simulink model "Properties_Controller_Tank1_Primitives"  (R2012b)
settings: Solver=FixedStepDiscrete  StartTime=0.0  StopTime=10.0  FixedStep=0.1  RelTol=1e-3
settings Model: Creator=Kerianne  LastModifiedBy=Kerianne
settings DataIOCC: SaveFormat=Structure
settings OptimizationCC: InlineParams=on

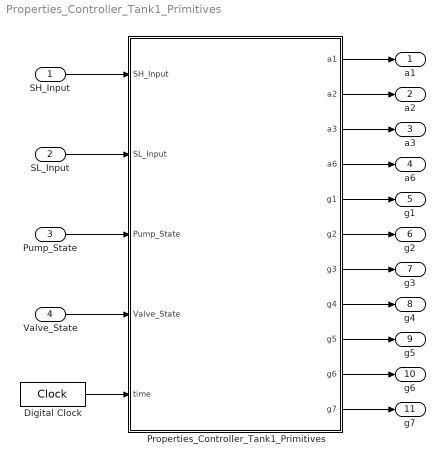
== system Properties_Controller_Tank1_Primitives ==
  SH_Input : Inport  OutDataTypeStr=double  SampleTime=0.1
  SL_Input : Inport  Port=2  OutDataTypeStr=double
  Pump_State : Inport  Port=3  OutDataTypeStr=double
  Valve_State : Inport  Port=4  OutDataTypeStr=double
  Digital Clock : DigitalClock  SampleTime=0.1
  Properties_Controller_Tank1_Primitives : MATLAB Function  TreatAsAtomicUnit=on
  a1 : Outport  OutDataTypeStr=boolean
  a2 : Outport  Port=2  OutDataTypeStr=boolean
  a3 : Outport  Port=3  OutDataTypeStr=boolean
  a6 : Outport  Port=4  OutDataTypeStr=boolean
  g1 : Outport  Port=5  OutDataTypeStr=boolean
  g2 : Outport  Port=6  OutDataTypeStr=boolean
  g3 : Outport  Port=7  OutDataTypeStr=boolean
  g4 : Outport  Port=8  OutDataTypeStr=boolean
  g5 : Outport  Port=9  OutDataTypeStr=boolean
  g6 : Outport  Port=10  OutDataTypeStr=boolean
  g7 : Outport  Port=11  OutDataTypeStr=boolean
  wires:
  SH_Input/1 -> Properties_Controller_Tank1_Primitives/1(SH_Input)
  Pump_State/1 -> Properties_Controller_Tank1_Primitives/3(Pump_State)
  Valve_State/1 -> Properties_Controller_Tank1_Primitives/4(Valve_State)
  SL_Input/1 -> Properties_Controller_Tank1_Primitives/2(SL_Input)
  Properties_Controller_Tank1_Primitives/9(g5) -> g5/1
  Properties_Controller_Tank1_Primitives/8(g4) -> g4/1
  Properties_Controller_Tank1_Primitives/7(g3) -> g3/1
  Properties_Controller_Tank1_Primitives/6(g2) -> g2/1
  Properties_Controller_Tank1_Primitives/5(g1) -> g1/1
  Properties_Controller_Tank1_Primitives/1(a1) -> a1/1
  Digital Clock/1 -> Properties_Controller_Tank1_Primitives/5(time)
  Properties_Controller_Tank1_Primitives/3(a3) -> a3/1
  Properties_Controller_Tank1_Primitives/2(a2) -> a2/1
  Properties_Controller_Tank1_Primitives/10(g6) -> g6/1
  Properties_Controller_Tank1_Primitives/11(g7) -> g7/1
  Properties_Controller_Tank1_Primitives/4(a6) -> a6/1

== matlab function Properties_Controller_Tank1_Primitives/Properties_Controller_Tank1_Primitives ==
  data: SH_Input input; a1 output; a2 output; a3 output; a6 output; g1 output; g2 output; g3 output; g4 output; g5 output; g6 output; SL_Input input; Pump_State input; Valve_State input; time input; g7 output
function [a1, a2, a3, a6, g1, g2, g3, g4, g5, g6, g7] = ...
    verification_condition(SH_Input, SL_Input, Pump_State, Valve_State, ...
    time)
% Tank 1 Controller Design Verifier
% Primitives Version
% Last Updated 23 Feb 2015
% Based on Controller Primitives Version

%% Persistent Variables
persistent pre_Valve_State
if isempty(pre_Valve_State)
    pre_Valve_State = 0;
    Valve_State = 0;
end
persistent pre_Pump_State
if isempty(pre_Pump_State)
    pre_Pump_State = 0;
    Pump_State = 0;
end


%% Assumptions
% assume "If the high sensor is true, then the low sensor is True"			
a1 = implies(SH_Input, SL_Input);
% assume "SH_Input is 0 (false) or 1(true)"
a2 = sensor_0_or_1(SH_Input);
% assume "SL_Input is 0 (false) or 1(true)"
a3 = sensor_0_or_1(SL_Input);
% assume "The Prev_Pump_State is the same as the output Pump_State in the
% previous step"
% assume "The Prev_Valve_State is the same as the output Valve_State in the 
% previous step" 
% assume "The Sensors are initially false"
a6 = sensors_initially_off(SH_Input, SL_Input, time);
%% Guarantees (Proof Objectives)
% guarantee "The pump is initially off"
g1 = pump_initially_off(pre_Pump_State, time);
% guarantee "The valve is initially closed"
g2 = valve_initially_closed(pre_Valve_State, time);	
% guarantee "After the initial time step, When SL_Input is False, the Pump shall be on and Valve shall be Closed" 
g3 = sl_input_false_cond(SL_Input, Pump_State, Valve_State, time);
% guarantee "When the SH_Input is true, the Pump shall be off and Valve shall be open"  
g4 = sh_input_true_cond(SH_Input, Pump_State, Valve_State);
% guarantee "When the SL_Input is True and the SH_Input is False, the Pump and Valve stay in their previous state"  
g5 = sl_input_true_sh_input_false_cond(SL_Input, SH_Input, Pump_State, Valve_State, pre_Pump_State, pre_Valve_State);
% assume "Pump State is 0 (off) or 1 (on)"
g6 = actuator_0_or_1(Pump_State);
% assume "Valve State is 0 (closed) or 1 (open)"
g7 = actuator_0_or_1(Valve_State);

pre_Pump_State = Pump_State;
pre_Valve_State = Valve_State;

%for a1
function c = implies(a,b)      
     c = ((not (a)) || b);
% for a2-a3
function result = sensor_0_or_1(sensor)
    result = (sensor == 1 | sensor == 0);
% for a6
function result = sensors_initially_off(SH_Input, SL_Input, time)
    UnderThisCondition = (time == 0.0);
    ResultShouldBe = (SH_Input == 0) && (SL_Input == 0);
    result = implies(UnderThisCondition, ResultShouldBe);
%for g1
function result = pump_initially_off(Pump_State, time)
    UnderThisCondition = (time == 0.0);
    ResultShouldBe = (Pump_State == 0);
    result = implies(UnderThisCondition, ResultShouldBe);
%for g2
function result = valve_initially_closed(Valve_State, time)
    UnderThisCondition = (time == 0.0);
    ResultShouldBe = (Valve_State == 0);
    result = implies(UnderThisCondition, ResultShouldBe);	
%for g3
function result = sl_input_false_cond(SL_Input, Pump_State, Valve_State, time) 
    UnderThisCondition = (SL_Input == 0) && (time > 0);
    ResultShouldBe = (Valve_State == 0) && (Pump_State == 1);
    result = implies(UnderThisCondition, ResultShouldBe); 
%for g4 
function result = sh_input_true_cond(SH_Input, Pump_State, Valve_State) 
    UnderThisCondition = (SH_Input == 1);
    ResultShouldBe = (Valve_State == 1) && (Pump_State == 0);
    result = implies(UnderThisCondition, ResultShouldBe); 
%for g5
function result = sl_input_true_sh_input_false_cond(SL_Input, SH_Input, Pump_State, Valve_State, pre_Pump_State, pre_Valve_State)
    UnderThisCondition = (SL_Input == 1) && (SH_Input == 0);
    ResultShouldBe = (Pump_State == pre_Pump_State) && (Valve_State == pre_Valve_State);
    result = implies(UnderThisCondition, ResultShouldBe);        
%for g6-g7
function result = actuator_0_or_1(actuator)
    result = (actuator == 0 | actuator == 1);


% % assume "Pump State is 0 (off) or 1 (on)"
% a4 = actuator_0_or_1(Pump_State);
% % assume "Valve State is 0 (closed) or 1 (open)"
% a5 = actuator_0_or_1(Valve_State); 
% % Additional Assumptions
% % assume "The Sensors are Initially False and the Pump is initially off"
% a6 = sensors_initially_false(SH_Input,SL_Input, Pump_State, time);
% %for a6-a7
% function result = actuator_0_or_1(actuator)
%     result = (actuator == false | actuator == true);
